simulink model "dubin"  (R2012b)
settings: Solver=ode45  StartTime=0.0  StopTime=10.0  RelTol=1e-3
settings Model: Creator=stsuei  LastModifiedBy=stsuei
settings DebuggingCC: SolverPrmCheckMsg=none

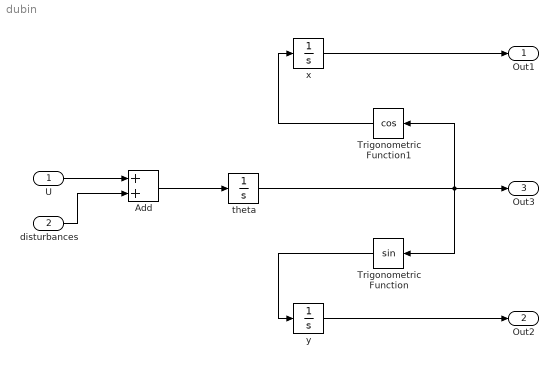
== system dubin ==
  U : Inport
  disturbances : Inport  Port=2
  Add : Sum
  Trigonometric Function : Trigonometry
  Trigonometric Function1 : Trigonometry  Operator=cos
  theta : Integrator
  x : Integrator
  y : Integrator
  Out1 : Outport
  Out2 : Outport  Port=2
  Out3 : Outport  Port=3
  wires:
  theta/1 -> Trigonometric Function/1, Trigonometric Function1/1, Out3/1
  y/1 -> Out2/1
  Trigonometric Function/1 -> y/1
  Trigonometric Function1/1 -> x/1
  x/1 -> Out1/1
  Add/1 -> theta/1
  disturbances/1 -> Add/2
  U/1 -> Add/1
